simulink model "MATLAB Simulink Model"  (R2020b)
settings: Solver=ode4  StartTime=0.0  StopTime=1  RelTol=1e-3
InitFcn:
  | clear;
  | clc;
  | 
  | %Motor Parameters
  | r1 = 1.405;
  | l1  = 0.005839;
  | r2 = 1.395;
  | l2 = 0.005839;
  | Lm = 0.1722;
  | 
  | %Motor Rated Values
  | Vrat = 400;
  | frat = 50;
  | 
  | x1 = 2*pi*frat*l1;
  | x2 = 2*pi*frat*l2;
  | Xm = 2*pi*frat*Lm;
  | Prat = 4*1000;
  | Nrat = 1430;
  | Ns = 120*frat/4;
  | nrat = Nrat*2*pi/60;
  | ns = Ns*2*pi/60;
  | srat = (Ns-Nrat)/Ns;
  | 
  | E1 = Vrat/sqrt(3); %phase voltage
  | IL = E1/( (r1 + (1i*x1) ) + ( ( (1i*x2) +(r2/srat) )*1i*Xm / ( (1i*Xm) + (1i*x2) + (r2/srat) ) ) );
  | E2 = E1 - (IL*(r1 + (1i*x1) ) );
  | Trat = (3/(ns))*srat*abs(E2)*abs(E2)*r2/((r2*r2) + (srat*srat*x2*x2));
  | %Trat = Prat/nrat;
  | 
  | %System Variables
  | Tsys = (1e-6);
  | Ts = (100e-6);
  | freq = 50;
  | 
  | m=1*freq/50;
  | %m = 1 * (freq/50);
  | Vbus = (400*sqrt(2)*2/sqrt(3)) / (1.15);
  | 
  | Vref = (Vbus*sqrt(3)/2) * m;
  | delay = Ts/Tsys;
  | 
  | % Motor Starting Parameters
  | inc_time = 0.1;
  | 
  | %Motor Loading time
  | load_time = 0.5;
  | 
  | %No. of Hybrid Zones
  | numzones = 3;
  | 
  | %Load ML model Weights
  | 
  | W1R_s1 = readmatrix('Regression Weights\W1_subnet1_tmp_odd_90.xlsx');
  | b1R_s1 = readmatrix('Regression Weights\b1_subnet1_tmp_odd_90.xlsx');
  | W1R_s2 = readmatrix('Regression Weights\W1_subnet2_tmp_odd_90.xlsx');
  | b1R_s2 = readmatrix('Regression Weights\b1_subnet2_tmp_odd_90.xlsx');
  | 
  | W2R = readmatrix('Regression Weights\W2_subnet_tmp_odd_90.xlsx');
  | b2R = readmatrix('Regression Weights\b2_subnet_tmp_odd_90.xlsx');
  | 
  | 
  | W1C_s1 = readmatrix('Classification Weights\W1_subnet1_tmp.xlsx');
  | b1C_s1 = readmatrix('Classification Weights\b1_subnet1_tmp.xlsx');
  | W1C_s2 = readmatrix('Classification Weights\W1_subnet2_tmp.xlsx');
  | b1C_s2 = readmatrix('Classification Weights\b1_subnet2_tmp.xlsx');
  | 
  | W2C = readmatrix('Classification Weights\W2_subnet_tmp.xlsx');
  | b2C = readmatrix('Classification Weights\b2_subnet_tmp.xlsx');
libraries: powerlib x72, simulink x55, powerlib_meascontrol x15, dspstat3 x11, dspsigops x1
(part 1 of 5)
settings Model: Creator=hp  LastModifiedBy=hp
settings DataIOCC: ReturnWorkspaceOutputs=off

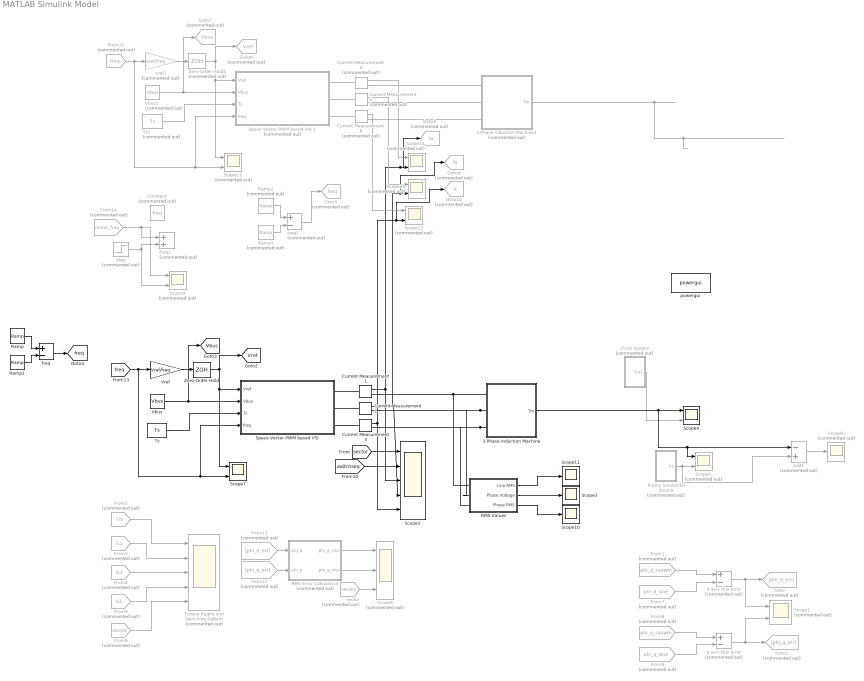
== system MATLAB Simulink Model ==
  15 Hz System : Subsystem  Commented=on
  3 Phase Induction Machine : Subsystem
  3 Phase Induction Machine1 : Subsystem  Commented=on
  Add1 : Sum  Commented=on  Inputs=-+
  Constant : Constant  Commented=on  Value=freq
  Current Measurement1 : powerlib/Measurements/Current Measurement  PhasorSimulation=off  OutputType=Complex  PSBequivalent=0
  Current Measurement2 : powerlib/Measurements/Current Measurement  PhasorSimulation=off  OutputType=Complex  PSBequivalent=0
  Current Measurement3 : powerlib/Measurements/Current Measurement  PhasorSimulation=off  OutputType=Complex  PSBequivalent=0
  Current Measurement4 : powerlib/Measurements/Current Measurement  Commented=on  PhasorSimulation=off  OutputType=Complex  PSBequivalent=0
  Current Measurement5 : powerlib/Measurements/Current Measurement  Commented=on  PhasorSimulation=off  OutputType=Complex  PSBequivalent=0
  Current Measurement6 : powerlib/Measurements/Current Measurement  Commented=on  PhasorSimulation=off  OutputType=Complex  PSBequivalent=0
  From1 : From  Commented=on  GotoTag=phi_d_svpwm  TagVisibility=global
  From11 : From  Commented=on  GotoTag=phi_d_err
  From12 : From  Commented=on  GotoTag=phi_q_err
  From14 : From  Commented=on  GotoTag=motor_freq  TagVisibility=global
  From15 : From  Commented=on  GotoTag=freq  TagVisibility=global
  From2 : From  Commented=on  GotoTag=Tm  TagVisibility=global
  From3 : From  Commented=on  GotoTag=G1  TagVisibility=global
  From4 : From  Commented=on  GotoTag=G3  TagVisibility=global
  From5 : From  Commented=on  GotoTag=G5  TagVisibility=global
  From6 : From  Commented=on  GotoTag=sector  TagVisibility=global
  From7 : From  Commented=on  GotoTag=phi_d_sine  TagVisibility=global
  From8 : From  Commented=on  GotoTag=phi_q_svpwm  TagVisibility=global
  From9 : From  Commented=on  GotoTag=phi_q_sine  TagVisibility=global
  Goto : Goto  Commented=on  GotoTag=phi_d_err
  Goto1 : Goto  Commented=on  GotoTag=phi_q_err
  Goto10 : Goto  Commented=on  GotoTag=ic  TagVisibility=global
  Goto5 : Goto  Commented=on  GotoTag=freq  TagVisibility=global
  Goto6 : Goto  Commented=on  GotoTag=Vref  TagVisibility=global
  Goto7 : Goto  Commented=on  GotoTag=Vbus  TagVisibility=global
  Goto8 : Goto  Commented=on  GotoTag=ia  TagVisibility=global
  Goto9 : Goto  Commented=on  GotoTag=ib  TagVisibility=global
  Purely Sinusoidal Source : Subsystem  Commented=on
  "RMS Error Calculation " : Subsystem  Commented=on
  RMS Values : Subsystem
  Ramp : simulink/Sources/Ramp  slope=freq/inc_time  start=0  InitialOutput=0
  Ramp1 : simulink/Sources/Ramp  slope=freq/inc_time  start=inc_time  InitialOutput=0
  Ramp2 : simulink/Sources/Ramp  Commented=on  slope=freq/inc_time  start=0  InitialOutput=0
  Ramp3 : simulink/Sources/Ramp  Commented=on  slope=freq/inc_time  start=inc_time  InitialOutput=0
  Scope{1,5,9,12..15} (7 alike) : Scope  Commented=on  NumInputPorts=2
  Scope10 : Scope
  Scope11 : Scope
  Scope2 : Scope  NumInputPorts=5
  Scope3 : Scope
  Scope4 : Scope  NumInputPorts=2
  Scope6 : Scope  Commented=on
  Scope7 : Scope  NumInputPorts=2
  Scope8 : Scope  Commented=on  NumInputPorts=3
  "Space Vector PWM based VSI " : Subsystem
  Space Vector PWM based VSI 1 : Subsystem  Commented=on
  Step : Step  Commented=on  Time=0.4  Before=50  After=10  SampleTime=Tsys
  Torque Ripple and Switching Pattern : Scope  Commented=on  NumInputPorts=5
  Ts : Constant  Value=Ts  SampleTime=Tsys
  Ts1 : Constant  Commented=on  Value=Ts  SampleTime=Tsys
  Vbus : Constant  Value=Vbus  SampleTime=Tsys
  Vbus1 : Constant  Commented=on  Value=Vbus  SampleTime=Tsys
  Vref : Gain  Gain=Vref/freq
  Vref1 : Gain  Commented=on  Gain=Vref/freq
  Zero-Order Hold : ZeroOrderHold  SampleTime=Ts
  Zero-Order Hold1 : ZeroOrderHold  Commented=on  SampleTime=Ts
  d axis flux error : Sum  Commented=on  Inputs=+-
  freq : Sum  Inputs=+-
  freq1 : Sum  Commented=on
  freq2 : Sum  Commented=on  Inputs=+-
  powergui : powerlib/powergui  Priority=1  SimulationMode=Discrete  SampleTime=1e-6  frequency=60  Iterations=50  frequencyindice=50  Pbase=100e6  ErrMax=1e-4  UnitsV=kV  UnitsW=MW  buscounter=0  FunctionMessages=off  echomessages=off  EnableUseOfTLC=off  CurrentSourceSwitches=off  DisableSnubberDevices=off  DisableRonSwitches=off  DisableVfSwitches=off  DisplayEquations=off  AutomaticDiscreteSolvers=off  SolverType=Tustin/Backward Euler (TBE)  Interpol=off  ExternalGateDelay=off  methode=off  Ts=100  x0status=blocks  SPID=on  SwTol=0  HookPort=off  NonlinearTolerance=1e-4  nMaxIteration=100  ContinueOnMaxIteration=off  RestoreLinks=warning  ResistiveCurrentMeasurement=off  Frange=[0:2:500]  Ylog=off  Xlog=on  ShowGrid=off  save=off  variable=ZData  structure=ScopeData4  ZoomFFT=off  StartTime=0.65  cycles=1  DisplayStyle=1  fundamental=50  FreqAxis=off  MaxFrequency=1000  frequencyindicesteady=1  RmsSteady=1  display=off
  q axis flux error : Sum  Commented=on  Inputs=+-
  sector : From  Commented=on  GotoTag=sector  TagVisibility=global
  tag scope: Vbus=global, Vref=global, freq=global
  wires:
  Ts/1 -> "Space Vector PWM based VSI "/3(Ts)
  Purely Sinusoidal Source/1(Tm) -> Add1/2, Scope5/2
  Add1/1 -> Scope6/1
  From2/1 -> Torque Ripple and Switching Pattern/1
  From6/1 -> Torque Ripple and Switching Pattern/5
  From7/1 -> d axis flux error/2
  From11/1 -> "RMS Error Calculation "/1(phi_d)
  From4/1 -> Torque Ripple and Switching Pattern/3
  From8/1 -> q axis flux error/1
  From3/1 -> Torque Ripple and Switching Pattern/2
  15 Hz System/1(Tm1) -> Scope4/2
  Ramp/1 -> freq/1
  sector/1 -> Scope8/3
  Current Measurement1/1 -> Goto8/1, Scope13/2, Scope2/3
  3 Phase Induction Machine/1(Tm) -> Scope5/1, Add1/1, Scope4/1
  From1/1 -> d axis flux error/1
  From12/1 -> "RMS Error Calculation "/2(phi_q)
  "RMS Error Calculation "/2(phi_q_rms) -> Scope8/2
  d axis flux error/1 -> Scope1/1, Goto/1
  "RMS Error Calculation "/1(phi_d_rms) -> Scope8/1
  From9/1 -> q axis flux error/2
  Vbus/1 -> [Vbus], "Space Vector PWM based VSI "/2(Vbus)
  From5/1 -> Torque Ripple and Switching Pattern/4
  q axis flux error/1 -> Scope1/2, Goto1/1
  Vref/1 -> Zero-Order Hold/1
  Current Measurement2/1 -> Goto9/1, Scope14/2, Scope2/4
  Current Measurement3/1 -> Scope2/5, Goto10/1, Scope15/2
  [sector] -> Scope2/1
  [switchseq] -> Scope2/2
  Zero-Order Hold/1 -> [Vref], "Space Vector PWM based VSI "/1(Vref), Scope7/1
  Ramp1/1 -> freq/2
  freq/1 -> [freq]
  [freq] -> "Space Vector PWM based VSI "/4(freq), Scope7/2, Vref/1
  Step/1 -> Scope9/2, freq1/2
  From14/1 -> Scope9/1, freq1/1
  From15/1 -> Vref1/1, Scope12/2, Space Vector PWM based VSI 1/4(freq)
  Zero-Order Hold1/1 -> Scope12/1, Space Vector PWM based VSI 1/1(Vref), Goto6/1
  Current Measurement6/1 -> Scope15/1
  Current Measurement5/1 -> Scope14/1
  Vref1/1 -> Zero-Order Hold1/1
  Vbus1/1 -> Space Vector PWM based VSI 1/2(Vbus), Goto7/1
  3 Phase Induction Machine1/1(Tm) -> ?
  Current Measurement4/1 -> Scope13/1
  Ts1/1 -> Space Vector PWM based VSI 1/3(Ts)
  Ramp3/1 -> freq2/2
  Ramp2/1 -> freq2/1
  freq2/1 -> Goto5/1
  RMS Values/1(Line RMS) -> Scope11/1
  RMS Values/2(Phase Voltage) -> Scope3/1
  RMS Values/3(Phase RMS) -> Scope10/1
  connections:
  3 Phase Induction Machine/LConn3 -- RMS Values/LConn3 -- Current Measurement3/RConn1
  Current Measurement1/LConn1 -- "Space Vector PWM based VSI "/RConn1
  Current Measurement2/LConn1 -- "Space Vector PWM based VSI "/RConn2
  Current Measurement3/LConn1 -- "Space Vector PWM based VSI "/RConn3
  Current Measurement5/RConn1 -- 3 Phase Induction Machine1/LConn2
  Current Measurement6/RConn1 -- 3 Phase Induction Machine1/LConn3
  Current Measurement4/RConn1 -- 3 Phase Induction Machine1/LConn1
  Current Measurement6/LConn1 -- Space Vector PWM based VSI 1/RConn3
  Current Measurement4/LConn1 -- Space Vector PWM based VSI 1/RConn1
  Current Measurement5/LConn1 -- Space Vector PWM based VSI 1/RConn2
  Current Measurement1/RConn1 -- 3 Phase Induction Machine/LConn1 -- RMS Values/LConn1
  3 Phase Induction Machine/LConn2 -- RMS Values/LConn2 -- Current Measurement2/RConn1

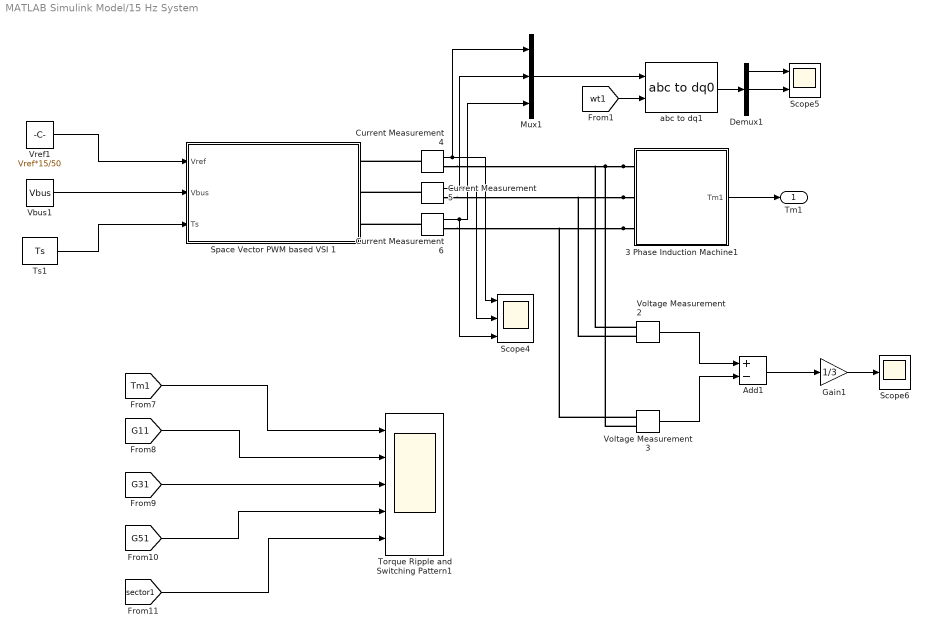
== system MATLAB Simulink Model/15 Hz System ==
  3 Phase Induction Machine1 : Subsystem
  Add1 : Sum  Inputs=+-
  Current Measurement4 : powerlib/Measurements/Current Measurement  PhasorSimulation=off  OutputType=Complex  PSBequivalent=0
  Current Measurement5 : powerlib/Measurements/Current Measurement  PhasorSimulation=off  OutputType=Complex  PSBequivalent=0
  Current Measurement6 : powerlib/Measurements/Current Measurement  PhasorSimulation=off  OutputType=Complex  PSBequivalent=0
  Demux1 : Demux  Outputs=3
  Gain1 : Gain  Gain=1/3
  Mux1 : Mux  Inputs=3
  Scope4 : Scope  NumInputPorts=3
  Scope5 : Scope  NumInputPorts=2
  Scope6 : Scope
  Space Vector PWM based VSI 1 : Subsystem
  Torque Ripple and Switching Pattern1 : Scope  NumInputPorts=5
  Ts1 : Constant  Value=Ts
  Vbus1 : Constant  Value=Vbus
  Voltage Measurement2 : powerlib/Measurements/Voltage Measurement  PhasorSimulation=off  OutputType=Complex  PSBequivalent=0
  Voltage Measurement3 : powerlib/Measurements/Voltage Measurement  PhasorSimulation=off  OutputType=Complex  PSBequivalent=0
  Vref1 : Constant  Value=Vref*15/50
  abc to dq1 : powerlib_meascontrol/Transformations/abc to dq0  Alignment=Aligned with phase A axis
  Tm1 : Outport
  wires:
  Current Measurement6/1 -> Mux1/3, Scope4/3
  Ts1/1 -> Space Vector PWM based VSI 1/3(Ts)
  [G51] -> Torque Ripple and Switching Pattern1/4
  Vref1/1 -> Space Vector PWM based VSI 1/1(Vref)
  [sector1] -> Torque Ripple and Switching Pattern1/5
  [wt1] -> abc to dq1/2
  abc to dq1/1 -> Demux1/1
  Current Measurement4/1 -> Scope4/1, Mux1/1
  [G31] -> Torque Ripple and Switching Pattern1/3
  Voltage Measurement3/1 -> Add1/2
  [G11] -> Torque Ripple and Switching Pattern1/2
  Current Measurement5/1 -> Mux1/2, Scope4/2
  Add1/1 -> Gain1/1
  [Tm1] -> Torque Ripple and Switching Pattern1/1
  Voltage Measurement2/1 -> Add1/1
  Demux1/2 -> Scope5/2
  Gain1/1 -> Scope6/1
  Demux1/1 -> Scope5/1
  Mux1/1 -> abc to dq1/1
  Vbus1/1 -> Space Vector PWM based VSI 1/2(Vbus)
  3 Phase Induction Machine1/1(Tm1) -> Tm1/1
  connections:
  3 Phase Induction Machine1/LConn3 -- Current Measurement6/RConn1 -- Voltage Measurement3/LConn1
  3 Phase Induction Machine1/LConn1 -- Current Measurement4/RConn1 -- Voltage Measurement2/LConn1 -- Voltage Measurement3/LConn2
  3 Phase Induction Machine1/LConn2 -- Current Measurement5/RConn1 -- Voltage Measurement2/LConn2
  Current Measurement5/LConn1 -- Space Vector PWM based VSI 1/RConn2
  Current Measurement6/LConn1 -- Space Vector PWM based VSI 1/RConn3
  Current Measurement4/LConn1 -- Space Vector PWM based VSI 1/RConn1

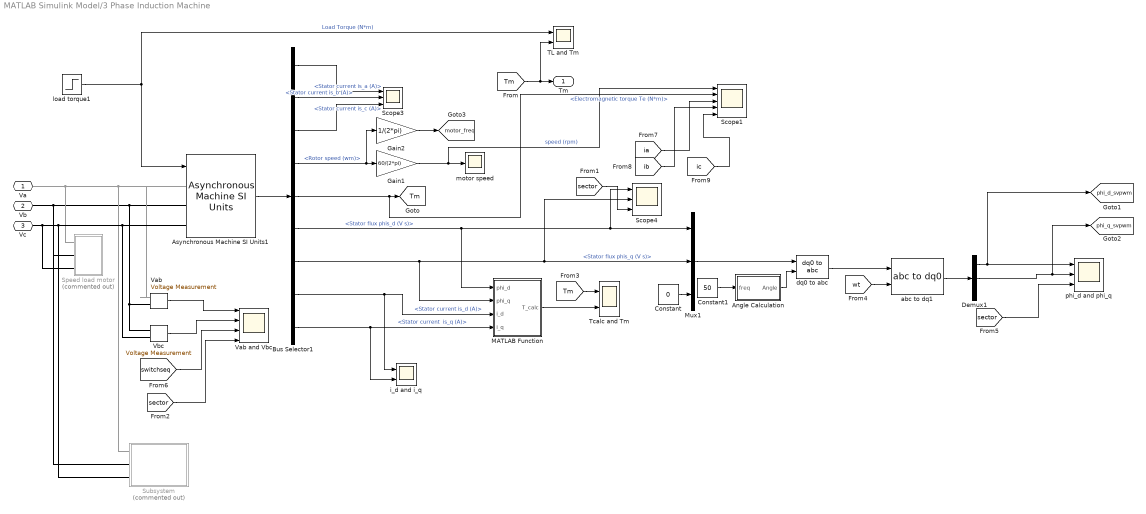
== system MATLAB Simulink Model/3 Phase Induction Machine ==
  Angle Calculation : Subsystem
  Asynchronous Machine SI Units1 : powerlib/Machines/Asynchronous Machine SI Units  RotorType=Squirrel-cage  PresetModel="15:  5.4 HP (4KW)   400 V  50Hz 1430 RPM"  MechanicalLoad=Torque Tm  ShowDetailedParameters=on  ReferenceFrame=Synchronous  Units=SI  MeasurementBus=off  NominalParameters=[4000 400 50]  Stator=[1.405 0.005839]  Rotor=[1.395 0.005839]  Cage1=[0.4155 0.002066]  Cage2=[0.4168 0.0003495]  Lm=0.1722  Mechanical=[0.0131 0.002985 2]  PolePairs=2  InitialConditions="[ 1,0   0,0,0   0,0,0 ]"  SimulateSaturation=off  Saturation=[14.03593122, 27.81365428, 53.79336849, 72.68890987, 97.98006896, 148.6815601, 215.7428561, 302.9841135, 428.7778367 ; 230, 322, 414, 460, 506, 552, 598, 644, 690]  LoadFlowParameters=1492000  TsPowergui=0  TsBlock=-1  IterativeModel=Trapezoidal non iterative  IterativeDiscreteModel=Trapezoidal non iterative  Pmec=0
  Bus Selector1 : BusSelector  OutputSignals="Stator measurements.Stator current is_a (A),Stator measurements.Stator current is_b (A),Stator measurements.Stator current is_c (A),Mechanical.Rotor speed (wm),Mechanical.Electromagnetic torque Te (N*m),Stator measurements.Stator flux phis_d (V s),Stator measurements.Stator flux phis_q (V s),Stator measurements.Stator current is_d (A),Stator measurements.Stator current  is_q (A)"
  Constant : Constant  Value=0
  Constant1 : Constant  Value=50  SampleTime=Tsys
  Demux1 : Demux  Outputs=3
  Gain1 : Gain  Gain=60/(2*pi)
  Gain2 : Gain  Gain=1/(2*pi)
  MATLAB Function : MATLAB Function  TreatAsAtomicUnit=on
  Mux1 : Mux  Inputs=3
  Scope1 : Scope  NumInputPorts=5
  Scope3 : Scope  NumInputPorts=3
  Scope4 : Scope  NumInputPorts=3
  Speed load motor : Subsystem  Commented=on
  Subsystem : Subsystem  Commented=on
  TL and Tm : Scope  NumInputPorts=2
  Tcalc and Tm : Scope  NumInputPorts=2
  Vab : powerlib/Measurements/Voltage Measurement  PhasorSimulation=off  OutputType=Complex  PSBequivalent=0
  Vab and Vbc : Scope  NumInputPorts=4
  Vbc : powerlib/Measurements/Voltage Measurement  PhasorSimulation=off  OutputType=Complex  PSBequivalent=0
  abc to dq1 : powerlib_meascontrol/Transformations/abc to dq0  Alignment=Aligned with phase A axis
  dq0 to abc : powerlib_meascontrol/Transformations/dq0 to abc  Alignment=90 degrees behind phase A axis
  i_d and i_q : Scope  NumInputPorts=2
  load torque1 : Step  Time=load_time  After=Trat  SampleTime=Tsys
  motor speed : Scope
  phi_d and phi_q : Scope  NumInputPorts=3
  Va : PMIOPort  Side=Left
  Vb : PMIOPort  Port=2  Side=Left
  Vc : PMIOPort  Port=3  Side=Left
  Tm : Outport
  tag scope: Tm=global, motor_freq=global, phi_d_svpwm=global, phi_q_svpwm=global
  wires:
  load torque1/1 -> TL and Tm/1, Asynchronous Machine SI Units1/1  "Load Torque (N*m)"
  Bus Selector1/4 -> Gain2/1, Gain1/1  "<Rotor speed (wm)>"
  Asynchronous Machine SI Units1/1 -> Bus Selector1/1
  Bus Selector1/2 -> Scope3/2  "<Stator current is_b (A)>"
  Bus Selector1/3 -> Scope3/3  "<Stator current is_c (A)>"
  Bus Selector1/1 -> Scope3/1  "<Stator current is_a (A)>"
  Bus Selector1/6 -> Mux1/1, Scope4/1, MATLAB Function/1(phi_d)  "<Stator flux phis_d (V s)>"
  Bus Selector1/7 -> Scope4/2, Mux1/2, MATLAB Function/2(phi_q)  "<Stator flux phis_q (V s)>"
  Gain1/1 -> Scope1/1, motor speed/1  "speed (rpm)"
  Bus Selector1/9 -> i_d and i_q/2, MATLAB Function/4(i_q)  "<Stator current  is_q (A)>"
  Bus Selector1/8 -> i_d and i_q/1, MATLAB Function/3(i_d)  "<Stator current is_d (A)>"
  MATLAB Function/1(T_calc) -> Tcalc and Tm/2
  Constant/1 -> Mux1/3
  Mux1/1 -> dq0 to abc/1
  Constant1/1 -> Angle Calculation/1(freq)
  Angle Calculation/1(Angle) -> dq0 to abc/2
  [Tm] -> Tcalc and Tm/1
  [sector] -> Scope4/3
  dq0 to abc/1 -> abc to dq1/1
  [wt] -> abc to dq1/2
  abc to dq1/1 -> Demux1/1
  Demux1/2 -> [phi_q_svpwm], phi_d and phi_q/2
  Demux1/1 -> phi_d and phi_q/1, [phi_d_svpwm]
  [sector] -> phi_d and phi_q/3
  Bus Selector1/5 -> Scope1/2, [Tm]  "<Electromagnetic torque Te (N*m)>"
  [Tm] -> Tm/1, TL and Tm/2
  Vbc/1 -> Vab and Vbc/2
  Vab/1 -> Vab and Vbc/1
  [sector] -> Vab and Vbc/4
  [switchseq] -> Vab and Vbc/3
  Gain2/1 -> [motor_freq]
  [ia] -> Scope1/3
  [ic] -> Scope1/5
  [ib] -> Scope1/4
  connections:
  Vab/LConn2 -- Subsystem/LConn2 -- Speed load motor/LConn2 -- Vb/RConn1 -- Asynchronous Machine SI Units1/LConn2 -- Vbc/LConn1
  Speed load motor/LConn1 -- Subsystem/LConn1 -- Vab/LConn1 -- Asynchronous Machine SI Units1/LConn1 -- Va/RConn1
  Vc/RConn1 -- Vbc/LConn2 -- Asynchronous Machine SI Units1/LConn3 -- Subsystem/LConn3 -- Speed load motor/LConn3

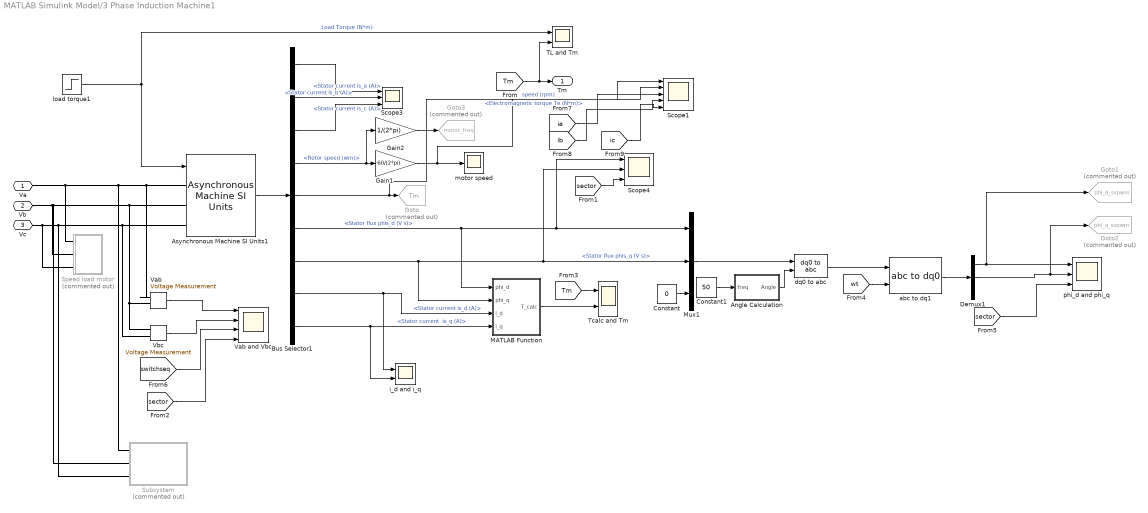
== system MATLAB Simulink Model/3 Phase Induction Machine1 ==
  Angle Calculation : Subsystem
  Asynchronous Machine SI Units1 : powerlib/Machines/Asynchronous Machine SI Units  RotorType=Squirrel-cage  PresetModel="15:  5.4 HP (4KW)   400 V  50Hz 1430 RPM"  MechanicalLoad=Torque Tm  ShowDetailedParameters=on  ReferenceFrame=Synchronous  Units=SI  MeasurementBus=off  NominalParameters=[4000 400 50]  Stator=[1.405 0.005839]  Rotor=[1.395 0.005839]  Cage1=[0.4155 0.002066]  Cage2=[0.4168 0.0003495]  Lm=0.1722  Mechanical=[0.0131 0.002985 2]  PolePairs=2  InitialConditions="[ 1,0   0,0,0   0,0,0 ]"  SimulateSaturation=off  Saturation=[14.03593122, 27.81365428, 53.79336849, 72.68890987, 97.98006896, 148.6815601, 215.7428561, 302.9841135, 428.7778367 ; 230, 322, 414, 460, 506, 552, 598, 644, 690]  LoadFlowParameters=1492000  TsPowergui=0  TsBlock=-1  IterativeModel=Trapezoidal non iterative  IterativeDiscreteModel=Trapezoidal non iterative  Pmec=0
  Bus Selector1 : BusSelector  OutputSignals="Stator measurements.Stator current is_a (A),Stator measurements.Stator current is_b (A),Stator measurements.Stator current is_c (A),Mechanical.Rotor speed (wm),Mechanical.Electromagnetic torque Te (N*m),Stator measurements.Stator flux phis_d (V s),Stator measurements.Stator flux phis_q (V s),Stator measurements.Stator current is_d (A),Stator measurements.Stator current  is_q (A)"
  Constant : Constant  Value=0
  Constant1 : Constant  Value=50  SampleTime=Tsys
  Demux1 : Demux  Outputs=3
  Gain1 : Gain  Gain=60/(2*pi)
  Gain2 : Gain  Gain=1/(2*pi)
  Goto : Goto  Commented=on  GotoTag=Tm  TagVisibility=global
  Goto1 : Goto  Commented=on  GotoTag=phi_d_svpwm  TagVisibility=global
  Goto2 : Goto  Commented=on  GotoTag=phi_q_svpwm  TagVisibility=global
  Goto3 : Goto  Commented=on  GotoTag=motor_freq  TagVisibility=global
  MATLAB Function : MATLAB Function  TreatAsAtomicUnit=on
  Mux1 : Mux  Inputs=3
  Scope1 : Scope  NumInputPorts=5
  Scope3 : Scope  NumInputPorts=3
  Scope4 : Scope  NumInputPorts=3
  Speed load motor : Subsystem  Commented=on
  Subsystem : Subsystem  Commented=on
  TL and Tm : Scope  NumInputPorts=2
  Tcalc and Tm : Scope  NumInputPorts=2
  Vab : powerlib/Measurements/Voltage Measurement  PhasorSimulation=off  OutputType=Complex  PSBequivalent=0
  Vab and Vbc : Scope  NumInputPorts=4
  Vbc : powerlib/Measurements/Voltage Measurement  PhasorSimulation=off  OutputType=Complex  PSBequivalent=0
  abc to dq1 : powerlib_meascontrol/Transformations/abc to dq0  Alignment=Aligned with phase A axis
  dq0 to abc : powerlib_meascontrol/Transformations/dq0 to abc  Alignment=90 degrees behind phase A axis
  i_d and i_q : Scope  NumInputPorts=2
  load torque1 : Step  Time=load_time  After=Trat  SampleTime=Tsys
  motor speed : Scope
  phi_d and phi_q : Scope  NumInputPorts=3
  Va : PMIOPort  Side=Left
  Vb : PMIOPort  Port=2  Side=Left
  Vc : PMIOPort  Port=3  Side=Left
  Tm : Outport
  wires:
  Gain2/1 -> Goto3/1
  [switchseq] -> Vab and Vbc/3
  [sector] -> Vab and Vbc/4
  Vab/1 -> Vab and Vbc/1
  Vbc/1 -> Vab and Vbc/2
  [Tm] -> TL and Tm/2, Tm/1
  Bus Selector1/5 -> Scope1/2, Goto/1  "<Electromagnetic torque Te (N*m)>"
  [sector] -> phi_d and phi_q/3
  Demux1/1 -> Goto1/1, phi_d and phi_q/1
  Demux1/2 -> phi_d and phi_q/2, Goto2/1
  abc to dq1/1 -> Demux1/1
  [wt] -> abc to dq1/2
  dq0 to abc/1 -> abc to dq1/1
  [sector] -> Scope4/3
  [Tm] -> Tcalc and Tm/1
  Angle Calculation/1(Angle) -> dq0 to abc/2
  Constant1/1 -> Angle Calculation/1(freq)
  Mux1/1 -> dq0 to abc/1
  Constant/1 -> Mux1/3
  MATLAB Function/1(T_calc) -> Tcalc and Tm/2
  Bus Selector1/8 -> MATLAB Function/3(i_d), i_d and i_q/1  "<Stator current is_d (A)>"
  Bus Selector1/9 -> MATLAB Function/4(i_q), i_d and i_q/2  "<Stator current  is_q (A)>"
  Gain1/1 -> Scope1/1, motor speed/1  "speed (rpm)"
  Bus Selector1/7 -> MATLAB Function/2(phi_q), Mux1/2, Scope4/2  "<Stator flux phis_q (V s)>"
  Bus Selector1/6 -> MATLAB Function/1(phi_d), Scope4/1, Mux1/1  "<Stator flux phis_d (V s)>"
  Bus Selector1/1 -> Scope3/1  "<Stator current is_a (A)>"
  Bus Selector1/3 -> Scope3/3  "<Stator current is_c (A)>"
  Bus Selector1/2 -> Scope3/2  "<Stator current is_b (A)>"
  Asynchronous Machine SI Units1/1 -> Bus Selector1/1
  Bus Selector1/4 -> Gain1/1, Gain2/1  "<Rotor speed (wm)>"
  load torque1/1 -> Asynchronous Machine SI Units1/1, TL and Tm/1  "Load Torque (N*m)"
  [ia] -> Scope1/3
  [ib] -> Scope1/4
  [ic] -> Scope1/5
  connections:
  Speed load motor/LConn3 -- Subsystem/LConn3 -- Asynchronous Machine SI Units1/LConn3 -- Vbc/LConn2 -- Vc/RConn1
  Va/RConn1 -- Asynchronous Machine SI Units1/LConn1 -- Vab/LConn1 -- Subsystem/LConn1 -- Speed load motor/LConn1
  Vbc/LConn1 -- Asynchronous Machine SI Units1/LConn2 -- Vb/RConn1 -- Speed load motor/LConn2 -- Subsystem/LConn2 -- Vab/LConn2

== system MATLAB Simulink Model/Purely Sinusoidal Source ==
  3 Phase Induction Machine1 : Subsystem
  Current Measurement4 : powerlib/Measurements/Current Measurement  PhasorSimulation=off  OutputType=Complex  PSBequivalent=0
  Current Measurement5 : powerlib/Measurements/Current Measurement  PhasorSimulation=off  OutputType=Complex  PSBequivalent=0
  Current Measurement6 : powerlib/Measurements/Current Measurement  PhasorSimulation=off  OutputType=Complex  PSBequivalent=0
  Demux : Demux  Outputs=3
  Mux : Mux  Inputs=3
  Scope2 : Scope  NumInputPorts=2
  Scope5 : Scope  NumInputPorts=3
  Three-Phase Source : powerlib/Electrical Sources/Three-Phase Source  InternalConnection=Yg  VoltagePhases=off  Voltage=Vref*sqrt(1/2)*1.15  PhaseAngle=89.10  Voltage_phases=[25e3 25e3 25e3]/sqrt(3)  PhaseAngles_phases=[0 -120 +120]  Frequency=freq  NonIdealSource=off  SpecifyImpedance=off  Resistance=0  Inductance=0  ShortCircuitLevel=100e6  BaseVoltage=0  XRratio=7  BusType=swing  Pref=10e3  Qref=0  Prefabc=[10e3, 10e3, 10e3]  Qrefabc=[0, 0, 0]  Qmin=-inf  Qmax=inf
  abc to dq0 : powerlib_meascontrol/Transformations/abc to dq0  Alignment=Aligned with phase A axis
  Tm : Outport
  wires:
  3 Phase Induction Machine1/1(Tm) -> Tm/1
  Demux/2 -> Scope2/2
  abc to dq0/1 -> Demux/1
  Demux/1 -> Scope2/1
  Current Measurement5/1 -> Scope5/2, Mux/2
  Current Measurement4/1 -> Mux/1, Scope5/1
  [wt] -> abc to dq0/2
  Mux/1 -> abc to dq0/1
  Current Measurement6/1 -> Mux/3, Scope5/3
  connections:
  Current Measurement4/RConn1 -- 3 Phase Induction Machine1/LConn1
  Current Measurement6/RConn1 -- 3 Phase Induction Machine1/LConn3
  Three-Phase Source/RConn1 -- Current Measurement4/LConn1
  Current Measurement5/RConn1 -- 3 Phase Induction Machine1/LConn2
  Three-Phase Source/RConn2 -- Current Measurement5/LConn1
  Three-Phase Source/RConn3 -- Current Measurement6/LConn1

== system MATLAB Simulink Model/RMS Error Calculation  ==
  phi_d : Inport
  phi_q : Inport  Port=2
  DC Blocker1 : dspsigops/DC Blocker  Commented=on  Algorithm=FIR  NormalizedBandwidth=0.001  Length=50  Order=6  SimulateUsing=Code generation
      settings: SourceProductName=DSP System Toolbox
  Moving RMS : dspstat3/Moving RMS  Method=Sliding window  ForgettingFactorPort=off  SpecifyWindowLength=on  WindowLength=int16(Ts/Tsys)  ForgettingFactor=0.9  SimulateUsing=Code generation
      settings: SourceProductBaseCode=DS
  Moving RMS1 : dspstat3/Moving RMS  Method=Sliding window  ForgettingFactorPort=off  SpecifyWindowLength=on  WindowLength=int16(Ts/Tsys)  ForgettingFactor=0.9  SimulateUsing=Code generation
      settings: SourceProductBaseCode=DS
  Scope13 : Scope  NumInputPorts=2
  Subsystem : Subsystem  Commented=on
  Zero-Order Hold1 : ZeroOrderHold  SampleTime=Ts
  Zero-Order Hold2 : ZeroOrderHold  SampleTime=Ts
  phi_d_rms : Outport
  phi_q_rms : Outport  Port=2
  wires:
  phi_d/1 -> Moving RMS/1, Subsystem/1(phi_d), Scope13/1
  Moving RMS/1 -> Zero-Order Hold1/1
  Moving RMS1/1 -> Zero-Order Hold2/1
  phi_q/1 -> Moving RMS1/1, Subsystem/2(phi_q), Scope13/2
  Zero-Order Hold2/1 -> phi_q_rms/1
  Zero-Order Hold1/1 -> phi_d_rms/1

== system MATLAB Simulink Model/RMS Values ==
  Add : Sum  Inputs=+-
  Gain : Gain  Gain=1/3
  RMS1 : powerlib_meascontrol/Measurements/RMS  TrueRMS=off  Freq=50  RMSInit=0  Ts=Tsys
  RMS2 : powerlib_meascontrol/Measurements/RMS  TrueRMS=off  Freq=freq  RMSInit=0  Ts=Tsys
  Voltage Measurement : powerlib/Measurements/Voltage Measurement  PhasorSimulation=off  OutputType=Complex  PSBequivalent=0
  Voltage Measurement1 : powerlib/Measurements/Voltage Measurement  PhasorSimulation=off  OutputType=Complex  PSBequivalent=0
  Va : PMIOPort  Side=Left
  Vb : PMIOPort  Port=2  Side=Left
  Vc : PMIOPort  Port=3  Side=Left
  Line RMS : Outport
  Phase Voltage : Outport  Port=2
  Phase RMS : Outport  Port=3
  wires:
  Gain/1 -> Phase Voltage/1, RMS1/1
  Voltage Measurement/1 -> RMS2/1, Add/1
  Voltage Measurement1/1 -> Add/2
  RMS1/1 -> Phase RMS/1
  Add/1 -> Gain/1
  RMS2/1 -> Line RMS/1
  connections:
  Voltage Measurement1/LConn2 -- Va/RConn1 -- Voltage Measurement/LConn1
  Voltage Measurement1/LConn1 -- Vc/RConn1
  Voltage Measurement/LConn2 -- Vb/RConn1

== system MATLAB Simulink Model/Space Vector PWM based VSI  ==
  Vref : Inport
  Vbus : Inport  Port=2
  Ts : Inport  Port=3
  freq : Inport  Port=4
  3 Phase VSI : Subsystem
  Gate Pulse Generator : Subsystem  Commented=on
  Gating Pulse Generator : Subsystem
  Scope1 : Scope  NumInputPorts=5
  Switching Times and Sector : Subsystem
  Van : PMIOPort  Side=Right
  Vbn : PMIOPort  Port=2  Side=Right
  Vcn : PMIOPort  Port=3  Side=Right
  tag scope: G1=global, G3=global, G5=global, sector=global
  wires:
  Vref/1 -> Switching Times and Sector/1(Vref)
  Ts/1 -> Switching Times and Sector/2(Ts)
  Vbus/1 -> Switching Times and Sector/3(Vbus)
  Switching Times and Sector/1(S1) -> Gating Pulse Generator/1(S1)
  Switching Times and Sector/2(S3) -> Gating Pulse Generator/2(S3)
  Switching Times and Sector/3(S5) -> Gating Pulse Generator/3(S5)
  Switching Times and Sector/4(sector) -> Gating Pulse Generator/4(sector), [sector]
  Switching Times and Sector/5(switchseq) -> Gating Pulse Generator/5(switchseq)
  Gating Pulse Generator/1(Gate 1 Pulse) -> [G1], 3 Phase VSI/1(Gate 1)
  Gating Pulse Generator/2(Gate 3 Pulse) -> [G3], 3 Phase VSI/2(Gate 3)
  Gating Pulse Generator/3(Gate 5 Pulse) -> [G5], 3 Phase VSI/3(Gate 5)
  [G1] -> Scope1/1
  [G3] -> Scope1/2
  [G5] -> Scope1/3
  [sector] -> Scope1/4
  [switchseq] -> Scope1/5
  freq/1 -> Switching Times and Sector/4(freq1)
  connections:
  Vbn/RConn1 -- 3 Phase VSI/RConn2
  Vcn/RConn1 -- 3 Phase VSI/RConn3
  3 Phase VSI/RConn1 -- Van/RConn1

== system MATLAB Simulink Model/Space Vector PWM based VSI 1 ==
  Vref : Inport
  Vbus : Inport  Port=2
  Ts : Inport  Port=3
  freq : Inport  Port=4
  3 Phase VSI : Subsystem
  Gate Pulse Generator : Subsystem  Commented=on
  Gating Pulse Generator : Subsystem
  Scope1 : Scope  NumInputPorts=5
  Switching Times and Sector : Subsystem
  Van : PMIOPort  Side=Right
  Vbn : PMIOPort  Port=2  Side=Right
  Vcn : PMIOPort  Port=3  Side=Right
  wires:
  freq/1 -> Switching Times and Sector/4(freq1)
  Gating Pulse Generator/3(Gate 5 Pulse) -> Scope1/5, 3 Phase VSI/3(Gate 5)
  Gating Pulse Generator/2(Gate 3 Pulse) -> Scope1/4, 3 Phase VSI/2(Gate 3)
  Gating Pulse Generator/1(Gate 1 Pulse) -> Scope1/3, 3 Phase VSI/1(Gate 1)
  Switching Times and Sector/5(switchseq) -> Gating Pulse Generator/5(switchseq), Scope1/2
  Switching Times and Sector/4(sector) -> Scope1/1, Gating Pulse Generator/4(sector)
  Switching Times and Sector/3(S5) -> Gating Pulse Generator/3(S5)
  Switching Times and Sector/2(S3) -> Gating Pulse Generator/2(S3)
  Switching Times and Sector/1(S1) -> Gating Pulse Generator/1(S1)
  Vbus/1 -> Switching Times and Sector/3(Vbus)
  Ts/1 -> Switching Times and Sector/2(Ts)
  Vref/1 -> Switching Times and Sector/1(Vref)
  connections:
  3 Phase VSI/RConn1 -- Van/RConn1
  Vcn/RConn1 -- 3 Phase VSI/RConn3
  Vbn/RConn1 -- 3 Phase VSI/RConn2

== system MATLAB Simulink Model/15 Hz System/3 Phase Induction Machine1 ==
  Asynchronous Machine SI Units1 : powerlib/Machines/Asynchronous Machine SI Units  RotorType=Squirrel-cage  PresetModel="15:  5.4 HP (4KW)   400 V  50Hz 1430 RPM"  MechanicalLoad=Torque Tm  ShowDetailedParameters=on  ReferenceFrame=Synchronous  Units=SI  MeasurementBus=off  NominalParameters=[4000 400 50]  Stator=[1.405 0.005839]  Rotor=[1.395 0.005839]  Cage1=[0.4155 0.002066]  Cage2=[0.4168 0.0003495]  Lm=0.1722  Mechanical=[0.0131 0.002985 2]  PolePairs=2  InitialConditions="[ 1,0   0,0,0   0,0,0 ]"  SimulateSaturation=off  Saturation=[14.03593122, 27.81365428, 53.79336849, 72.68890987, 97.98006896, 148.6815601, 215.7428561, 302.9841135, 428.7778367 ; 230, 322, 414, 460, 506, 552, 598, 644, 690]  LoadFlowParameters=1492000  TsPowergui=0  TsBlock=-1  IterativeModel=Trapezoidal non iterative  IterativeDiscreteModel=Trapezoidal non iterative  Pmec=0
  Bus Selector1 : BusSelector  OutputSignals=Stator measurements.Stator current is_a (A),Stator measurements.Stator current is_b (A),Stator measurements.Stator current is_c (A),Mechanical.Rotor speed (wm),Mechanical.Electromagnetic torque Te (N*m),Stator measurements.Stator flux phis_d (V s),Stator measurements.Stator flux phis_q (V s)
  Demux : Demux  Outputs=3
  Gain2 : Gain  Gain=4/2
  Mux : Mux  Inputs=3
  Scope{1,4,6,8} (4 alike) : Scope  NumInputPorts=2
  Scope2 : Scope
  Scope3 : Scope  NumInputPorts=3
  Voltage Measurement1 : powerlib/Measurements/Voltage Measurement  PhasorSimulation=off  OutputType=Complex  PSBequivalent=0
  Voltage Measurement3 : powerlib/Measurements/Voltage Measurement  PhasorSimulation=off  OutputType=Complex  PSBequivalent=0
  Voltage Measurement4 : powerlib/Measurements/Voltage Measurement  PhasorSimulation=off  OutputType=Complex  PSBequivalent=0
  abc to dq0 : powerlib_meascontrol/Transformations/abc to dq0  Alignment=Aligned with phase A axis
  load torque1 : Step  Time=0.5  After=20  SampleTime=0
  Va : PMIOPort  Side=Left
  Vb : PMIOPort  Port=2  Side=Left
  Vc : PMIOPort  Port=3  Side=Left
  Tm1 : Outport
  tag scope: Tm1=global
  wires:
  Voltage Measurement3/1 -> Mux/1, Scope8/1
  load torque1/1 -> Scope6/2, Asynchronous Machine SI Units1/1  "Load Torque (N*m)"
  Gain2/1 -> Scope2/1  "speed (rad/s)"
  Bus Selector1/4 -> Gain2/1  "<Rotor speed (wm)>"
  Asynchronous Machine SI Units1/1 -> Bus Selector1/1
  Bus Selector1/2 -> Scope3/2  "<Stator current is_b (A)>"
  Bus Selector1/3 -> Scope3/3  "<Stator current is_c (A)>"
  Voltage Measurement4/1 -> Mux/2, Scope8/2
  Bus Selector1/5 -> [Tm1], Tm1/1, Scope6/1  "<Electromagnetic torque Te (N*m)>"
  Bus Selector1/1 -> Scope3/1  "<Stator current is_a (A)>"
  [wt1] -> abc to dq0/2
  Mux/1 -> abc to dq0/1
  Demux/2 -> Scope1/2
  Demux/1 -> Scope1/1
  abc to dq0/1 -> Demux/1
  Voltage Measurement1/1 -> Mux/3
  Bus Selector1/6 -> Scope4/1  "<Stator flux phis_d (V s)>"
  Bus Selector1/7 -> Scope4/2  "<Stator flux phis_q (V s)>"
  connections:
  Asynchronous Machine SI Units1/LConn2 -- Voltage Measurement4/LConn1 -- Voltage Measurement3/LConn2 -- Vb/RConn1
  Voltage Measurement4/LConn2 -- Voltage Measurement1/LConn1 -- Asynchronous Machine SI Units1/LConn3 -- Vc/RConn1
  Voltage Measurement3/LConn1 -- Voltage Measurement1/LConn2 -- Va/RConn1 -- Asynchronous Machine SI Units1/LConn1

== system MATLAB Simulink Model/15 Hz System/Space Vector PWM based VSI 1 ==
  Vref : Inport
  Vbus : Inport  Port=2
  Ts : Inport  Port=3
  3 Phase VSI : Subsystem
  Gate Pulse Generator : Subsystem
  Switching Times and Sector : Subsystem
  Va : PMIOPort  Side=Right
  Vb : PMIOPort  Port=2  Side=Right
  Vc : PMIOPort  Port=3  Side=Right
  tag scope: G11=global, G31=global, G51=global
  wires:
  Gate Pulse Generator/2(Gate 3 Pulse) -> 3 Phase VSI/2(Gate 3), [G31]
  Gate Pulse Generator/1(Gate 1 Pulse) -> [G11], 3 Phase VSI/1(Gate 1)
  Gate Pulse Generator/3(Gate 5 Pulse) -> 3 Phase VSI/3(Gate 5), [G51]
  Vref/1 -> Switching Times and Sector/1(Vref)
  Ts/1 -> Switching Times and Sector/2(Ts)
  Vbus/1 -> Switching Times and Sector/3(Vbus)
  Switching Times and Sector/1("S1, S3, S5, sector") -> Gate Pulse Generator/1("S1, S3, S5, sector")
  connections:
  Vb/RConn1 -- 3 Phase VSI/RConn2
  Vc/RConn1 -- 3 Phase VSI/RConn3
  Va/RConn1 -- 3 Phase VSI/RConn1

== system MATLAB Simulink Model/3 Phase Induction Machine/Angle Calculation ==
  freq : Inport
  Delay : Delay  DelayLength=1  InitialCondition=0  UseCircularBuffer=on
  Gain1 : Gain  Gain=Tsys
  MATLAB Function : MATLAB Function  TreatAsAtomicUnit=on
  Scope : Scope
  Zero-Order Hold : ZeroOrderHold  SampleTime=Ts
  w : Gain  Gain=2*pi
  Angle : Outport
  wires:
  freq/1 -> w/1, Scope/1
  Gain1/1 -> MATLAB Function/2(wTs)
  Zero-Order Hold/1 -> Angle/1
  Delay/1 -> MATLAB Function/1(wold)
  MATLAB Function/1(wnew) -> Delay/1, Zero-Order Hold/1
  w/1 -> Gain1/1

== system MATLAB Simulink Model/3 Phase Induction Machine/Speed load motor ==
  Asynchronous Machine SI Units3 : powerlib/Machines/Asynchronous Machine SI Units  RotorType=Squirrel-cage  PresetModel="15:  5.4 HP (4KW)   400 V  50Hz 1430 RPM"  MechanicalLoad=Speed w  ShowDetailedParameters=on  ReferenceFrame=Synchronous  Units=SI  MeasurementBus=off  NominalParameters=[4000 400 50]  Stator=[1.405 0.005839]  Rotor=[1.395 0.005839]  Cage1=[0.4155 0.002066]  Cage2=[0.4168 0.0003495]  Lm=0.1722  Mechanical=[0.0131 0.002985 2]  PolePairs=2  InitialConditions="[ 1,0   0,0,0   0,0,0 ]"  SimulateSaturation=off  Saturation=[14.03593122, 27.81365428, 53.79336849, 72.68890987, 97.98006896, 148.6815601, 215.7428561, 302.9841135, 428.7778367 ; 230, 322, 414, 460, 506, 552, 598, 644, 690]  LoadFlowParameters=1492000  TsPowergui=0  TsBlock=-1  IterativeModel=Trapezoidal non iterative  IterativeDiscreteModel=Trapezoidal non iterative  Pmec=0
  Bus Selector3 : BusSelector  OutputSignals=Stator measurements.Stator current is_a (A),Stator measurements.Stator current is_b (A),Stator measurements.Stator current is_c (A),Mechanical.Rotor speed (wm),Mechanical.Electromagnetic torque Te (N*m),Stator measurements.Stator flux phis_d (V s),Stator measurements.Stator flux phis_q (V s)
  Gain2 : Gain  Gain=60/(2*pi)
  Gain3 : Gain  Gain=60/(2*pi)
  Scope10 : Scope
  Scope5 : Scope  NumInputPorts=2
  Scope7 : Scope  NumInputPorts=3
  Scope9 : Scope  NumInputPorts=3
  speed : Step  Time=load_time  Before=ns  After=nrat  SampleTime=0
  Va : PMIOPort  Side=Left
  Vb : PMIOPort  Port=2  Side=Left
  Vc : PMIOPort  Port=3  Side=Left
  wires:
  [sector] -> Scope9/3
  speed/1 -> Asynchronous Machine SI Units3/1, Gain3/1  "Angular speed (rad/s)"
  Bus Selector3/5 -> Scope10/1  "<Electromagnetic torque Te (N*m)>"
  Bus Selector3/1 -> Scope7/1  "<Stator current is_a (A)>"
  Gain2/1 -> Scope5/2  "speed (rpm)"
  Asynchronous Machine SI Units3/1 -> Bus Selector3/1
  Bus Selector3/6 -> Scope9/1  "<Stator flux phis_d (V s)>"
  Bus Selector3/3 -> Scope7/3  "<Stator current is_c (A)>"
  Gain3/1 -> Scope5/1  "speed (rpm)"
  Bus Selector3/7 -> Scope9/2  "<Stator flux phis_q (V s)>"
  Bus Selector3/4 -> Gain2/1  "<Rotor speed (wm)>"
  Bus Selector3/2 -> Scope7/2  "<Stator current is_b (A)>"
  connections:
  Asynchronous Machine SI Units3/LConn2 -- Vb/RConn1
  Asynchronous Machine SI Units3/LConn1 -- Va/RConn1
  Vc/RConn1 -- Asynchronous Machine SI Units3/LConn3

== system MATLAB Simulink Model/3 Phase Induction Machine/Subsystem ==
  Add : Sum  Inputs=+-
  Add1 : Sum  Inputs=+-
  Add2 : Sum  Inputs=+-
  Clock : Clock
  Demux : Demux  Outputs=3
  Mux : Mux  Inputs=3
  To Workspace : ToWorkspace  VariableName=Valpha  SampleTime=-1
  To Workspace1 : ToWorkspace  VariableName=Vbeta  SampleTime=-1
  To Workspace2 : ToWorkspace  VariableName=time_out1  SampleTime=-1
  Va : Gain  Gain=1/3
  Vab : powerlib/Measurements/Voltage Measurement  PhasorSimulation=off  OutputType=Complex  PSBequivalent=0
  Vb : Gain  Gain=1/3
  Vbc : powerlib/Measurements/Voltage Measurement  PhasorSimulation=off  OutputType=Complex  PSBequivalent=0
  Vc : Gain  Gain=1/3
  Vca : powerlib/Measurements/Voltage Measurement  PhasorSimulation=off  OutputType=Complex  PSBequivalent=0
  XY Graph : simulink/Sinks/XY Graph  Commented=on  xmin=-500  xmax=500  ymin=-500  ymax=500  st=-1
  abc to Alpha-Beta-Zero : powerlib_meascontrol/Transformations/abc to Alpha-Beta-Zero
  a : PMIOPort  Tag=PMCPort  Side=Left
  b : PMIOPort  Tag=PMCPort  Port=2  Side=Left
  c : PMIOPort  Tag=PMCPort  Port=3  Side=Left
  wires:
  Mux/1 -> abc to Alpha-Beta-Zero/1
  Add/1 -> Va/1
  Vab/1 -> Add2/2, Add/1
  Vbc/1 -> Add1/1, Add/2
  Add1/1 -> Vb/1
  Vca/1 -> Add2/1, Add1/2
  Add2/1 -> Vc/1
  Va/1 -> Mux/1
  Vb/1 -> Mux/2
  Vc/1 -> Mux/3
  abc to Alpha-Beta-Zero/1 -> Demux/1
  Demux/1 -> XY Graph/1, To Workspace/1
  Demux/2 -> XY Graph/2, To Workspace1/1
  Clock/1 -> To Workspace2/1
  connections:
  Vab/LConn2 -- b/RConn1 -- Vbc/LConn1
  Vbc/LConn2 -- c/RConn1 -- Vca/LConn1
  a/RConn1 -- Vca/LConn2 -- Vab/LConn1

== system MATLAB Simulink Model/3 Phase Induction Machine1/Angle Calculation ==
  freq : Inport
  Delay : Delay  DelayLength=1  InitialCondition=0  UseCircularBuffer=on
  Gain1 : Gain  Gain=Tsys
  MATLAB Function : MATLAB Function  TreatAsAtomicUnit=on
  Scope : Scope
  Zero-Order Hold : ZeroOrderHold  SampleTime=Ts
  w : Gain  Gain=2*pi
  Angle : Outport
  wires:
  w/1 -> Gain1/1
  MATLAB Function/1(wnew) -> Zero-Order Hold/1, Delay/1
  Delay/1 -> MATLAB Function/1(wold)
  Zero-Order Hold/1 -> Angle/1
  Gain1/1 -> MATLAB Function/2(wTs)
  freq/1 -> Scope/1, w/1

== system MATLAB Simulink Model/3 Phase Induction Machine1/Speed load motor ==
  Asynchronous Machine SI Units3 : powerlib/Machines/Asynchronous Machine SI Units  RotorType=Squirrel-cage  PresetModel="15:  5.4 HP (4KW)   400 V  50Hz 1430 RPM"  MechanicalLoad=Speed w  ShowDetailedParameters=on  ReferenceFrame=Synchronous  Units=SI  MeasurementBus=off  NominalParameters=[4000 400 50]  Stator=[1.405 0.005839]  Rotor=[1.395 0.005839]  Cage1=[0.4155 0.002066]  Cage2=[0.4168 0.0003495]  Lm=0.1722  Mechanical=[0.0131 0.002985 2]  PolePairs=2  InitialConditions="[ 1,0   0,0,0   0,0,0 ]"  SimulateSaturation=off  Saturation=[14.03593122, 27.81365428, 53.79336849, 72.68890987, 97.98006896, 148.6815601, 215.7428561, 302.9841135, 428.7778367 ; 230, 322, 414, 460, 506, 552, 598, 644, 690]  LoadFlowParameters=1492000  TsPowergui=0  TsBlock=-1  IterativeModel=Trapezoidal non iterative  IterativeDiscreteModel=Trapezoidal non iterative  Pmec=0
  Bus Selector3 : BusSelector  OutputSignals=Stator measurements.Stator current is_a (A),Stator measurements.Stator current is_b (A),Stator measurements.Stator current is_c (A),Mechanical.Rotor speed (wm),Mechanical.Electromagnetic torque Te (N*m),Stator measurements.Stator flux phis_d (V s),Stator measurements.Stator flux phis_q (V s)
  Gain2 : Gain  Gain=60/(2*pi)
  Gain3 : Gain  Gain=60/(2*pi)
  Scope10 : Scope
  Scope5 : Scope  NumInputPorts=2
  Scope7 : Scope  NumInputPorts=3
  Scope9 : Scope  NumInputPorts=3
  speed : Step  Time=load_time  Before=ns  After=nrat  SampleTime=0
  Va : PMIOPort  Side=Left
  Vb : PMIOPort  Port=2  Side=Left
  Vc : PMIOPort  Port=3  Side=Left
  wires:
  Bus Selector3/2 -> Scope7/2  "<Stator current is_b (A)>"
  Bus Selector3/4 -> Gain2/1  "<Rotor speed (wm)>"
  Bus Selector3/7 -> Scope9/2  "<Stator flux phis_q (V s)>"
  Gain3/1 -> Scope5/1  "speed (rpm)"
  Bus Selector3/3 -> Scope7/3  "<Stator current is_c (A)>"
  Bus Selector3/6 -> Scope9/1  "<Stator flux phis_d (V s)>"
  Asynchronous Machine SI Units3/1 -> Bus Selector3/1
  Gain2/1 -> Scope5/2  "speed (rpm)"
  Bus Selector3/1 -> Scope7/1  "<Stator current is_a (A)>"
  Bus Selector3/5 -> Scope10/1  "<Electromagnetic torque Te (N*m)>"
  speed/1 -> Gain3/1, Asynchronous Machine SI Units3/1  "Angular speed (rad/s)"
  [sector] -> Scope9/3
  connections:
  Vc/RConn1 -- Asynchronous Machine SI Units3/LConn3
  Asynchronous Machine SI Units3/LConn1 -- Va/RConn1
  Asynchronous Machine SI Units3/LConn2 -- Vb/RConn1

== system MATLAB Simulink Model/3 Phase Induction Machine1/Subsystem ==
  Add : Sum  Inputs=+-
  Add1 : Sum  Inputs=+-
  Add2 : Sum  Inputs=+-
  Clock : Clock
  Demux : Demux  Outputs=3
  Mux : Mux  Inputs=3
  To Workspace : ToWorkspace  VariableName=Valpha  SampleTime=-1
  To Workspace1 : ToWorkspace  VariableName=Vbeta  SampleTime=-1
  To Workspace2 : ToWorkspace  VariableName=time_out1  SampleTime=-1
  Va : Gain  Gain=1/3
  Vab : powerlib/Measurements/Voltage Measurement  PhasorSimulation=off  OutputType=Complex  PSBequivalent=0
  Vb : Gain  Gain=1/3
  Vbc : powerlib/Measurements/Voltage Measurement  PhasorSimulation=off  OutputType=Complex  PSBequivalent=0
  Vc : Gain  Gain=1/3
  Vca : powerlib/Measurements/Voltage Measurement  PhasorSimulation=off  OutputType=Complex  PSBequivalent=0
  XY Graph : simulink/Sinks/XY Graph  Commented=on  xmin=-500  xmax=500  ymin=-500  ymax=500  st=-1
  abc to Alpha-Beta-Zero : powerlib_meascontrol/Transformations/abc to Alpha-Beta-Zero
  a : PMIOPort  Tag=PMCPort  Side=Left
  b : PMIOPort  Tag=PMCPort  Port=2  Side=Left
  c : PMIOPort  Tag=PMCPort  Port=3  Side=Left
  wires:
  Clock/1 -> To Workspace2/1
  Demux/2 -> To Workspace1/1, XY Graph/2
  Demux/1 -> To Workspace/1, XY Graph/1
  abc to Alpha-Beta-Zero/1 -> Demux/1
  Vc/1 -> Mux/3
  Vb/1 -> Mux/2
  Va/1 -> Mux/1
  Add2/1 -> Vc/1
  Vca/1 -> Add1/2, Add2/1
  Add1/1 -> Vb/1
  Vbc/1 -> Add/2, Add1/1
  Vab/1 -> Add/1, Add2/2
  Add/1 -> Va/1
  Mux/1 -> abc to Alpha-Beta-Zero/1
  connections:
  Vab/LConn1 -- Vca/LConn2 -- a/RConn1
  Vca/LConn1 -- c/RConn1 -- Vbc/LConn2
  Vbc/LConn1 -- b/RConn1 -- Vab/LConn2

== system MATLAB Simulink Model/Purely Sinusoidal Source/3 Phase Induction Machine1 ==
  Asynchronous Machine SI Units1 : powerlib/Machines/Asynchronous Machine SI Units  RotorType=Squirrel-cage  PresetModel="15:  5.4 HP (4KW)   400 V  50Hz 1430 RPM"  MechanicalLoad=Torque Tm  ShowDetailedParameters=on  ReferenceFrame=Synchronous  Units=SI  MeasurementBus=off  NominalParameters=[4000 400 50]  Stator=[1.405 0.005839]  Rotor=[1.395 0.005839]  Cage1=[0.4155 0.002066]  Cage2=[0.4168 0.0003495]  Lm=0.1722  Mechanical=[0.0131 0.002985 2]  PolePairs=2  InitialConditions="[ 1,0   0,0,0   0,0,0 ]"  SimulateSaturation=off  Saturation=[14.03593122, 27.81365428, 53.79336849, 72.68890987, 97.98006896, 148.6815601, 215.7428561, 302.9841135, 428.7778367 ; 230, 322, 414, 460, 506, 552, 598, 644, 690]  LoadFlowParameters=1492000  TsPowergui=0  TsBlock=-1  IterativeModel=Trapezoidal non iterative  IterativeDiscreteModel=Trapezoidal non iterative  Pmec=0
  Bus Selector1 : BusSelector  OutputSignals=Stator measurements.Stator current is_a (A),Stator measurements.Stator current is_b (A),Stator measurements.Stator current is_c (A),Mechanical.Rotor speed (wm),Mechanical.Electromagnetic torque Te (N*m),Stator measurements.Stator flux phis_d (V s),Stator measurements.Stator flux phis_q (V s)
  Demux : Demux  Outputs=3
  Gain2 : Gain  Gain=60/(2*pi)
  Mux : Mux  Inputs=3
  Scope{1,4,6,8} (4 alike) : Scope  NumInputPorts=2
  Scope2 : Scope
  Scope3 : Scope  NumInputPorts=3
  Voltage Measurement1 : powerlib/Measurements/Voltage Measurement  PhasorSimulation=off  OutputType=Complex  PSBequivalent=0
  Voltage Measurement3 : powerlib/Measurements/Voltage Measurement  PhasorSimulation=off  OutputType=Complex  PSBequivalent=0
  Voltage Measurement4 : powerlib/Measurements/Voltage Measurement  PhasorSimulation=off  OutputType=Complex  PSBequivalent=0
  abc to dq0 : powerlib_meascontrol/Transformations/abc to dq0  Alignment=Aligned with phase A axis
  load torque1 : Step  Time=load_time  After=Trat  SampleTime=0
  Va : PMIOPort  Side=Left
  Vb : PMIOPort  Port=2  Side=Left
  Vc : PMIOPort  Port=3  Side=Left
  Tm : Outport
  tag scope: phi_d_sine=global, phi_q_sine=global
  wires:
  Voltage Measurement3/1 -> Mux/1, Scope8/1
  load torque1/1 -> Scope6/2, Asynchronous Machine SI Units1/1  "Load Torque (N*m)"
  Gain2/1 -> Scope2/1  "speed (rad/s)"
  Bus Selector1/4 -> Gain2/1  "<Rotor speed (wm)>"
  Asynchronous Machine SI Units1/1 -> Bus Selector1/1
  Bus Selector1/2 -> Scope3/2  "<Stator current is_b (A)>"
  Bus Selector1/3 -> Scope3/3  "<Stator current is_c (A)>"
  Voltage Measurement4/1 -> Mux/2, Scope8/2
  Bus Selector1/5 -> Scope6/1, Tm/1  "<Electromagnetic torque Te (N*m)>"
  Bus Selector1/1 -> Scope3/1  "<Stator current is_a (A)>"
  [wt] -> abc to dq0/2
  Mux/1 -> abc to dq0/1
  Demux/2 -> Scope1/2
  Demux/1 -> Scope1/1
  abc to dq0/1 -> Demux/1
  Voltage Measurement1/1 -> Mux/3
  Bus Selector1/6 -> Scope4/1, [phi_d_sine]  "<Stator flux phis_d (V s)>"
  Bus Selector1/7 -> Scope4/2, [phi_q_sine]  "<Stator flux phis_q (V s)>"
  connections:
  Asynchronous Machine SI Units1/LConn2 -- Voltage Measurement4/LConn1 -- Voltage Measurement3/LConn2 -- Vb/RConn1
  Voltage Measurement4/LConn2 -- Voltage Measurement1/LConn1 -- Asynchronous Machine SI Units1/LConn3 -- Vc/RConn1
  Voltage Measurement3/LConn1 -- Voltage Measurement1/LConn2 -- Va/RConn1 -- Asynchronous Machine SI Units1/LConn1

== system MATLAB Simulink Model/RMS Error Calculation /Subsystem ==
  phi_d : Inport
  phi_q : Inport  Port=2
  Constant : Constant  Value=Ts
  Constant1 : Constant  Value=Tsys
  Delay{,1..3} (4 alike) : Delay  DelayLength=1
  Gain1 : Gain  Gain=1/Ts
  Gain2 : Gain  Gain=1/Ts
  MATLAB Function : MATLAB Function  TreatAsAtomicUnit=on
  MATLAB Function1 : MATLAB Function  TreatAsAtomicUnit=on
  Zero-Order Hold : ZeroOrderHold  SampleTime=Ts
  Zero-Order Hold2 : ZeroOrderHold  SampleTime=Ts
  drms : Sqrt  SaturateOnIntegerOverflow=on
  qrms : Sqrt  SaturateOnIntegerOverflow=on
  Out1 : Outport
  Out2 : Outport  Port=2
  wires:
  Zero-Order Hold/1 -> Gain1/1
  MATLAB Function/2(curr_it_num) -> Delay1/1
  MATLAB Function/1(phi_d_rms) -> Delay/1, Zero-Order Hold/1
  MATLAB Function1/1(phi_q_rms) -> Zero-Order Hold2/1, Delay2/1
  Delay1/1 -> MATLAB Function/2(prev_it_num)
  Constant/1 -> MATLAB Function1/2(Ts), MATLAB Function/4(Ts)
  qrms/1 -> Out2/1
  MATLAB Function1/2(curr_it_num) -> Delay3/1
  Gain1/1 -> drms/1
  Delay2/1 -> MATLAB Function1/4("phi_q_rms ")
  Delay/1 -> MATLAB Function/1("phi_d_rms ")
  Gain2/1 -> qrms/1
  Zero-Order Hold2/1 -> Gain2/1
  Constant1/1 -> MATLAB Function/5(Tsys), MATLAB Function1/1(Tsys)
  Delay3/1 -> MATLAB Function1/5(prev_it_num)
  drms/1 -> Out1/1
  phi_q/1 -> MATLAB Function1/3(phi_q)
  phi_d/1 -> MATLAB Function/3(phi_d)
